simulink model "ALL_JP360_DBW_V6_5_1103"  (R2022a)
settings: Solver=FixedStepAuto  StartTime=0.0  StopTime=inf  FixedStep=0.01  RelTol=1e-3  EnableMultiTasking=on
model workspace (MAT data in the model file):
  g = 9.8
undefined symbols (not defined in the file or in its folder): canChannel, delta_v_p, IPM_Line_C0, IPM_Line_C1, IPM_Line_C2, IPM_Line_C3, M, M_p, MRR_ObjDistX, MRR_ObjDistY, MRR_ObjFusionCamID, MRR_ObjFusionSig, MRR_ObjID, MRR_ObjRelVelX, MRR_ObjRelVelY, MRR_ObjType, MRR_ObjUpdFlg, none, obj_vaild, untracktime, V, videoinput
libraries: canfdmsglib x230, canfdlib x76, slpidlib x24, simulink x18, dspstat3 x14, ctrlSharedLib x1, simulink_extras x1, imaqlib x1, realtime_pacer_lib x1, dspvision x1, visionsinks x1
(part 54 of 55)

== stateflow chart ALL_JP360_DBW_V6_5_1103/ACC_Control/ACC_FUNCTION/acc_stateflow/Chart2 ==
  settings: executeAtInitialization=1
  state total
    en:active_flg=0;set_flg=0;
    state a_set [parallel]
      settings: executionOrder=2
      state active
        state out
          en:set_speed_out=fcc(ABS_VehSpdLgt);
        state in
        state out_two
          en:set_speed_out=set_speed_in;
          du:set_speed_out=set_speed_in;
        (default) -> in
        in -> out [order 1] : [hasChangedFrom(SWM_ACCSet,0)]
        out -> out_two : [hasChangedFrom(SWM_ACCSet,0)||hasChangedFrom(SWM_ACCResume,0)]
        in -> out_two [order 2] : [hasChangedFrom(SWM_ACCResume,0)]
      state not_active
      state nomal_active
        du:set_speed_out=set_speed_in;
      not_active -> active [order 1] : [active_flg==1&&set_flg==1]
      (default) -> not_active
      active -> not_active : [active_flg~=1||set_flg~=1]
      nomal_active -> not_active : [active_flg==0]
      not_active -> nomal_active [order 2] : [active_flg==1&&set_flg==0]
    state acc [parallel]
      settings: executionOrder=1
      state NONE
      state INIT
        en:ACC_Status=0;flg=0;flg_quit=0;active_flg=0;
      note: set_resume=0:未激活
          | set_resume=1:按set激活
          | set_resume=2:按resume激活
      state AFTER_INIT
        state OFF
          en:ACC_Status=0;
          en:set_speed_out=0;
          en:flg=0;
          en:active_flg=0;set_flg=0;
        state STANDBY
          en:ACC_Status=2;
          en:active_flg=0;
        state PASSIVE
          en:ACC_Status=1;
          en:active_flg=0;
        state OVERRIDE
          en:ACC_Status=5;
          en:active_flg=0;
        state ACTIVE
          en:flg=flg+1;active_flg=1;
          state ACTIVE_CONTROL
            en:ACC_Status=3;
          state STAND_ACTIVE
            en:ACC_Status=6;
            en:three_s=1;
            en:flg_quit=flg_quit+1;
            du:flg_quit=flg_quit+1;
            state OFF
              y_stop=0;
            state ON
              en:y_stop=y_stop+1;
              du:y_stop=y_stop+1;
            (default) -> total.acc.AFTER_INIT.ACTIVE.STAND_ACTIVE.OFF
            total.acc.AFTER_INIT.ACTIVE.STAND_ACTIVE.OFF -> ON
          state STAND_WAIT
            en:ACC_Status=6;
            en:three_s=0;
            en:flg_quit=flg_quit+1;
            du:flg_quit=flg_quit+1;
          (default) -> ACTIVE_CONTROL
          STAND_WAIT -> ACTIVE_CONTROL [order 2] : [hasChangedFrom(SWM_ACCResume,1)&&EMS_BrkPedalStasus==0&&DriveOff==1&&SRS_SBR_Driver==0&&BCM_DoorStsFrntLe==1&&BCM_DoorStsFrntRi==1&&BCM_DoorStsRearLe==1&&BCM_DoorStsRearRi==1]{flg_quit=0}
          ACTIVE_CONTROL -> STAND_ACTIVE [order 1] : [ESP_VehicleStandstill==1&&SRS_SBR_Driver==0&&EMS_BrkPedalStasus==0&&DriveOff==0]
          STAND_ACTIVE -> ACTIVE_CONTROL [order 1] : [SRS_SBR_Driver==0&&EMS_BrkPedalStasus==0&&DriveOff==1]{flg_quit=0}
          STAND_ACTIVE -> STAND_WAIT [order 2] : [y_stop>=300]
          STAND_WAIT -> STAND_ACTIVE [order 1] : [hasChangedFrom(SWM_ACCResume,1)&&SRS_SBR_Driver==0&&EMS_BrkPedalStasus==0&&DriveOff==0]
        (default) -> total.acc.AFTER_INIT.OFF
        total.acc.AFTER_INIT.OFF -> STANDBY [order 2] : [hasChangedFrom(SWM_ACCSwitch,0)&&SWM_ACCSwitch~=2&&~(EMS_BrkPedalStasus==1||ESP_EPBStatus==1||ESP_EPBStatus==3||BCM_Mechanical_Hand_Brake==2||TCU_GearSelectorReq~=5||ABS_VehSpdDirection==1||BCM_DoorStsFrntLe==2||BCM_DoorStsFrntRi==2||BCM_DoorStsRearLe==2||BCM_DoorStsRearRi==2||BCM_EnginehoodSts==2||SRS_SBR_Driver==2)]
        STANDBY -> total.acc.AFTER_INIT.OFF [order 2] : [hasChangedFrom(SWM_ACCSwitch,0)&&SWM_ACCSwitch~=2]
        ACTIVE -> total.acc.AFTER_INIT.OFF [order 2] : [hasChangedFrom(SWM_ACCSwitch,0)&&SWM_ACCSwitch==2]{set_flg=0}
        total.acc.AFTER_INIT.OFF -> PASSIVE [order 1] : [hasChangedFrom(SWM_ACCSwitch,0)&&SWM_ACCSwitch~=2&&(EMS_BrkPedalStasus==1||ESP_EPBStatus==1||ESP_EPBStatus==3||BCM_Mechanical_Hand_Brake==2||TCU_GearSelectorReq~=5||ABS_VehSpdDirection==1||BCM_DoorStsFrntLe==2||BCM_DoorStsFrntRi==2||BCM_DoorStsRearLe==2||BCM_DoorStsRearRi==2||BCM_EnginehoodSts==2||SRS_SBR_Driver==2)]
        PASSIVE -> total.acc.AFTER_INIT.OFF [order 2] : [hasChangedFrom(SWM_ACCSwitch,0)&&SWM_ACCSwitch~=2]
        OVERRIDE -> total.acc.AFTER_INIT.OFF [order 3] : [hasChangedFrom(SWM_ACCSwitch,0)&&SWM_ACCSwitch==2]
        PASSIVE -> STANDBY [order 1] : [~(EMS_BrkPedalStasus==1||ESP_EPBStatus==1||ESP_EPBStatus==3||BCM_Mechanical_Hand_Brake==2||TCU_GearSelectorReq~=5||ABS_VehSpdDirection==1||BCM_DoorStsFrntLe==2||BCM_DoorStsFrntRi==2||BCM_DoorStsRearLe==2||BCM_DoorStsRearRi==2||BCM_EnginehoodSts==2||SRS_SBR_Driver==2)]
        (junction 53) -> PASSIVE
        STANDBY -> PASSIVE [order 1] : [EMS_BrkPedalStasus==1||ESP_EPBStatus==1||ESP_EPBStatus==3||BCM_Mechanical_Hand_Brake==2||TCU_GearSelectorReq~=5||ABS_VehSpdDirection==1||BCM_DoorStsFrntLe==2||BCM_DoorStsFrntRi==2||BCM_DoorStsRearLe==2||BCM_DoorStsRearRi==2||BCM_EnginehoodSts==2||SRS_SBR_Driver==2]
        (junction 140) -> (junction 53) : [(hasChangedFrom(SWM_ACCSwitch,0)&&SWM_ACCSwitch~=2)||ESP_EPBStatus==1||ESP_EPBStatus==3||BCM_Mechanical_Hand_Brake==2||TCU_GearSelectorReq~=5||ABS_VehSpdDirection==1||BCM_DoorStsFrntLe==2||BCM_DoorStsFrntRi==2||BCM_DoorStsRearLe==2||BCM_DoorStsRearRi==2||BCM_EnginehoodSts==2||SRS_SBR_Driver==2||flg_quit>=18000]{flg_quit=0,set_flg=0}
        ACTIVE_CONTROL -> (junction 53) [order 2] : [(hasChangedFrom(SWM_ACCSwitch,0)&&SWM_ACCSwitch~=2)||EMS_BrkPedalStasus==1||ESP_EPBStatus==1||ESP_EPBStatus==3||BCM_Mechanical_Hand_Brake==2||TCU_GearSelectorReq~=5||ABS_VehSpdDirection==1||BCM_DoorStsFrntLe==2||BCM_DoorStsFrntRi==2||BCM_DoorStsRearLe==2||BCM_DoorStsRearRi==2||BCM_EnginehoodSts==2||SRS_SBR_Driver==2]{set_flg=0}
        STANDBY -> ACTIVE [order 3] : [hasChangedFrom(SWM_ACCSet,0)&&~(EMS_BrkPedalStasus==1||ESP_EPBStatus==1||ESP_EPBStatus==3||BCM_Mechanical_Hand_Brake==2||TCU_GearSelectorReq~=5||ABS_VehSpdDirection==1||BCM_DoorStsFrntLe==2||BCM_DoorStsFrntRi==2||BCM_DoorStsRearLe==2||BCM_DoorStsRearRi==2||BCM_EnginehoodSts==2||SRS_SBR_Driver==2)&&(EMS_AccRAWPedalRatio==0||EMS_AccRAWPedalRatio==255)]{set_speed_out=fcc(ABS_VehSpdLgt)}
        STANDBY -> ACTIVE [order 4] : [(hasChangedFrom(SWM_ACCResume,0)&&flg~=0)&&~(EMS_BrkPedalStasus==1||ESP_EPBStatus==1||ESP_EPBStatus==3||BCM_Mechanical_Hand_Brake==2||TCU_GearSelectorReq~=5||ABS_VehSpdDirection==1||BCM_DoorStsFrntLe==2||BCM_DoorStsFrntRi==2||BCM_DoorStsRearLe==2||BCM_DoorStsRearRi==2||BCM_EnginehoodSts==2||SRS_SBR_Driver==2)&&(EMS_AccRAWPedalRatio==0||EMS_AccRAWPedalRatio==255)]
        OVERRIDE -> PASSIVE [order 2] : [(hasChangedFrom(SWM_ACCSwitch,0)&&SWM_ACCSwitch~=2)||EMS_BrkPedalStasus==1||ESP_EPBStatus==1||ESP_EPBStatus==3||BCM_Mechanical_Hand_Brake==2||TCU_GearSelectorReq~=5||ABS_VehSpdDirection==1||BCM_DoorStsFrntLe==2||BCM_DoorStsFrntRi==2||BCM_DoorStsRearLe==2||BCM_DoorStsRearRi==2||BCM_EnginehoodSts==2||SRS_SBR_Driver==2]
        OVERRIDE -> ACTIVE [order 1] : [EMS_IndicatedDriverOverride==0]{set_flg=1}
        ACTIVE -> OVERRIDE [order 1] : [EMS_IndicatedDriverOverride==1]{set_flg=0}
        STAND_WAIT -> (junction 140) [order 3]
        STAND_ACTIVE -> (junction 140) [order 3]
      state FALURE_REVERSIBLE
        en:ACC_Status=7;
        en:active_flg=0;
      state FALURE_IRREVERSIBLE
        en:ACC_Status=7;
        en:active_flg=0;
      (default) -> NONE
      NONE -> INIT : [BCM_PowerModeInvalid==0&&BCM_PowerMode==2&&ESP_EspEnableSts==1&&EPS_EPSPAMSts~=7&&EMS_IndicatedEngError==0&&MRR_HWFail==0&&IPM_SensorState==0]
      INIT -> AFTER_INIT
      AFTER_INIT -> FALURE_REVERSIBLE [order 1] : [acc_state_sw==1]
      FALURE_REVERSIBLE -> AFTER_INIT [order 1] : [acc_state_sw==0]
      FALURE_REVERSIBLE -> FALURE_IRREVERSIBLE [order 2] : [acc_state_sw==2||ESP_EspEnableSts==0||EPS_EPSPAMSts==7||EMS_IndicatedEngError==1||MRR_HWFail==1||IPM_SensorState==4]
      AFTER_INIT -> FALURE_IRREVERSIBLE [order 2] : [acc_state_sw==2||ESP_EspEnableSts==0||EPS_EPSPAMSts==7||EMS_IndicatedEngError==1||MRR_HWFail==1||IPM_SensorState==4]
  data: y function_output; VehSpdLgt function_input; SWM_ACCSwitch input; SWM_ACCSet input; SWM_ACCResume input; BCM_DoorStsFrntLe input; BCM_DoorStsFrntRi input; BCM_DoorStsRearLe input; BCM_DoorStsRearRi input; BCM_PowerModeInvalid input; BCM_PowerMode input; BCM_Mechanical_Hand_Brake input; BCM_EnginehoodSts input; IPM_SensorState input; MRR_HWFail input; SRS_SBR_Driver input; EMS_IndicatedEngError input; EMS_AccRAWPedalRatio input; EMS_BrkPedalStasus input; EPS_EPSPAMSts input; TCU_GearSelectorReq input; ESP_EPBStatus input; ESP_EspEnableSts input; ABS_VehSpdDirection input; ESP_AvhActive input; ESP_VehicleStandstill input; DriveOff input; acc_state_sw input; ACC_Status output int8; flg local; set_speed_in input; ABS_VehSpdLgt input; EMS_IndicatedDriverOverride input; set_speed_out output uint8; three_s output; y_stop local; flg_quit local; active_flg local; set_flg local
  function y=fcc(VehSpdLgt):
    | function y=fcc(VehSpdLgt)
    |  
    | if VehSpdLgt <=uint8(30)
    |     y=uint8(30);
    | else
    |     y=VehSpdLgt;
    | end
    | 
    | end

== matlab function ALL_JP360_DBW_V6_5_1103/ACC_Control/ACC_FUNCTION/Subsystem2/Limit/a2m_表达式_标定表/MATLAB Function ==
  data: delta_v input; y output; p1 input; p2 input
function y = fcn(delta_v,p1,p2)
    if delta_v < 1 && delta_v > -0.05
        y = single(p1);
    elseif delta_v <=-0.05
        y = single(p2);
    else
        y=single(0);
    end
end

== matlab function ALL_JP360_DBW_V6_5_1103/ACC_Control/ACC_FUNCTION/Subsystem2/ACC_model/CC_module/MATLAB Function ==
  data: acc_in input; delta_v input; acc_out output; dec_in input; dec_out output
function [acc_out, dec_out] = fcn(acc_in,delta_v, dec_in)
    if delta_v > -2.5
        acc_out = acc_in;
%         if delta_v >-0.1
%             dec_out = single(0);
%         else
%             if dec_in < 0
%                 dec_in = dec_in + single(0.05);
%                 dec_out = dec_in;
%             else
                dec_out = single(0);
%             end
%         end
    else
        acc_out = single(0);
        dec_out = dec_in;
    end
end

== matlab function ALL_JP360_DBW_V6_5_1103/ACC_Control/ACC_FUNCTION/Subsystem2/Limit/MATLAB Function ==
  data: u input; y1 output; data input; y2 output
function [y1,y2] = fcn(u, data)
%此函数的功能为：当err_v在(-1,0)时，输出-10nm；(-2,-1)时，输出扭矩-30nm；
%err_v小于等于-2时，输出PID计算的减速度；
y1=single(0);
y2=single(0);
if -1<u&&u<0
    y1=single(-10);
elseif -2<u&&u<=-1
    y1=single(-30);
elseif u<=-2
    y2=single(data);
else
    y1=single(0);
    y2=single(0);
end

== stateflow chart ALL_JP360_DBW_V6_5_1103/button/ACCset/ACC_button/Subsystem4/Chart1 ==
  state ON
    en:y=y+t;
    du:y=y+t;
  state OFF
    y=0;
  (default) -> (junction 1)
  (junction 1) -> OFF [order 2]
  (junction 1) -> ON [order 1] : [u1==3]
  OFF -> ON : [u1==3]
  ON -> OFF : [u1~=3]
  data: y output uint16; t input uint16; u1 input int8

== stateflow chart ALL_JP360_DBW_V6_5_1103/DCLC1/DCLC状态机/Chart1 ==
  state OFF
    en:
    count = 0;
  state ON
    en:
    count = count + 1;
    du:
    count = count + 1;
  (default) -> OFF
  OFF -> ON : [condition == 1]
  ON -> OFF : [condition == 0]
  data: condition input; count output

== stateflow chart ALL_JP360_DBW_V6_5_1103/ACC_Control/ACC_FUNCTION/Subsystem2/override/Chart2 ==
  settings: executeAtInitialization=1
  state ON
  state OFF
  (default) -> OFF
  OFF -> ON : status{u1=1}
  ON -> OFF : mode{u1=0}
  data: u1 output
  events: status input EITHER_EDGE_EVENT; mode input EITHER_EDGE_EVENT

== matlab function ALL_JP360_DBW_V6_5_1103/DCLC1/AngleSaftyLimitedCal ==
  data: a input single; angle_limited output single; L input single; V input single; angle input single
function angle_limited= fcn(a,L,V,angle)
if abs(V) > 19.5
    a = single(0.8);
end
angle_max = atan(a*L/V/V)*16*57.3;
if angle > angle_max
    angle_limited = angle_max;
elseif angle < -angle_max
        angle_limited = -angle_max;
else
    angle_limited = angle;
end

if angle_limited > single(20)
    angle_limited = single(20);
elseif angle_limited < -20
    angle_limited = single(-20);
end

end

== matlab function ALL_JP360_DBW_V6_5_1103/LKA_Control/LKA_Cal/LKAControlerl/MATLAB Function ==
  data: LKA_status input int8; err input; ang_rate output single; LKA_sta data_store_memory; t_ca data_store_memory; sta_change data_store_memory
function ang_rate = fcn(LKA_status,err)

global LKA_sta;
global t_ca;
global sta_change;

if LKA_sta==1 && LKA_status ==4
    sta_change = int8(1);
end
if LKA_status ==4 && sta_change == 1
    t_ca = t_ca +int8(1);
    ang_rate = single(2);
    if err <0.15 || t_ca >300
        sta_change = int8(0);
        t_ca = int8(0);
        ang_rate = single(25);
    end
else
    sta_change = int8(0);
    t_ca =int8(0);
    ang_rate = single(25);
end

end

== stateflow chart ALL_JP360_DBW_V6_5_1103/button/ACCset/ACC_button/Subsystem4/Chart2 ==
  state init
    state ON
      y=true;
    state OFF
      y=false;
    init -> (junction 1)
    (default) -> (junction 1)
    (junction 1) -> OFF [order 2]
    (junction 1) -> ON [order 1] : [u1>=20]
  (default) -> init
  data: y output boolean; u1 input uint16

== stateflow chart ALL_JP360_DBW_V6_5_1103/button/ACCset/ACC_button/Subsystem3/Chart ==
  state ON
    en:y=y+t;
    du:y=y+t;
  state OFF
    y=0;
  (default) -> (junction 1)
  (junction 1) -> OFF [order 2]
  (junction 1) -> ON [order 1] : [u1==1]
  OFF -> ON : [u1==1]
  ON -> OFF : [u1==0]
  data: y output uint16; t input; u1 input

== stateflow chart ALL_JP360_DBW_V6_5_1103/button/ACCset/ACC_button/Subsystem3/Chart10 ==
  state init
    state ON1
      en:y=1;
    state ON
      en:y=floor(u1/80)+1;
    state OFF
      y=0;
    init -> (junction 1)
    (default) -> (junction 1)
    (junction 1) -> OFF [order 3]
    (junction 1) -> ON [order 1] : [u1>=80]
    (junction 1) -> ON1 [order 2] : [u1>=4&&u1<80]
  (default) -> init
  data: y output single; u1 input single

== stateflow chart ALL_JP360_DBW_V6_5_1103/button/ACCset/ACC_button/accsetv2 ==
  state s1
    speedout=false;
  state s
    speedout=speed;
  (default) -> s1
  s1 -> s : [accs==3]
  s -> s1 : [accs~=3]
  data: speedout output boolean; accs input; speed input boolean

== stateflow chart ALL_JP360_DBW_V6_5_1103/button/ACCset/ACC_button/Subsystem1/Chart ==
  state ON
    en:y=y+t;
    du:y=y+t;
  state OFF
    y=0;
  (default) -> (junction 1)
  (junction 1) -> OFF [order 2]
  (junction 1) -> ON [order 1] : [u1==1]
  OFF -> ON : [u1==1]
  ON -> OFF : [u1==0]
  data: y output uint16; t input; u1 input

== stateflow chart ALL_JP360_DBW_V6_5_1103/button/ACCset/ACC_button/Subsystem1/Chart10 ==
  state init
    state ON1
      en:y=1;
    state ON
      en:y=fix(u1/80)+1;
    state OFF
      y=0;
    init -> (junction 1)
    (default) -> (junction 1)
    (junction 1) -> OFF [order 3]
    (junction 1) -> ON [order 1] : [u1>=80]
    (junction 1) -> ON1 [order 2] : [u1>=4&&u1<80]
  (default) -> init
  data: y output single; u1 input single

== stateflow chart ALL_JP360_DBW_V6_5_1103/button/ACCset/ACC_button/accsetv1 ==
  state s1
    speedout=false;
  state s
    speedout=speed;
  (default) -> s1
  s1 -> s : [accs==3]
  s -> s1 : [accs~=3]
  data: speedout output boolean; accs input; speed input boolean

== stateflow chart ALL_JP360_DBW_V6_5_1103/button/ACCset/ACC_button/Chart1 ==
  state s
    state start1
      a=speed;
    state pluss
      en:a=floor(speed/10)*10+10;
    state pluss1
      en:a=speed+1;
    state minn1
      en:a=ceil(speed/10)*10-10;
    state minn
      en:a=speed-1;
    s -> (junction 54)
    (default) -> start1
    (junction 54) -> start1 [order 5]
    (junction 54) -> minn [order 3] : [min==1]
    (junction 54) -> minn1 [order 1] : [min>=2]
    (junction 54) -> pluss [order 2] : [plus>=2]
    (junction 54) -> pluss1 [order 4] : [plus==1]
  (default) -> s
  data: a output; plus input; min input; speed input
  events: event input RISING_EDGE_EVENT

== stateflow chart ALL_JP360_DBW_V6_5_1103/button/ACCset/ACC_button/Chart2 ==
  state s
    state s
    state pluss1
      speedout=150;
    state minn1
      speedout=30;
    state minn
      speedout=speed;
    state minn2 [commented out]
      speedout=0;
    s -> (junction 54)
    (default) -> s.s
    (junction 54) -> s.s [order 4]
    (junction 54) -> minn [order 2] : [speed>=30&&speed<=150]
    (junction 54) -> minn2 [commented out] : [speed==0]
    (junction 54) -> minn1 [order 1] : [speed<=30&&speed>=0]
    (junction 54) -> pluss1 [order 3] : [speed>150]
  (default) -> s
  data: speedout output uint8; speed input

== stateflow chart ALL_JP360_DBW_V6_5_1103/button/ACCset/ACC_button/Subsystem2/Chart ==
  state ON
    en:y=y+t;
    du:y=y+t;
  state OFF
    y=0;
  (default) -> (junction 1)
  (junction 1) -> OFF [order 2]
  (junction 1) -> ON [order 1] : [u1==1]
  OFF -> ON : [u1==1]
  ON -> OFF : [u1==0]
  data: y output uint16; t input; u1 input

== stateflow chart ALL_JP360_DBW_V6_5_1103/button/ACCset/ACC_button/Subsystem2/Chart10 ==
  state init
    state ON1
      en:y=1;
    state ON
      en:y=fix(u1/80)+1;
    state OFF
      y=0;
    init -> (junction 1)
    (default) -> (junction 1)
    (junction 1) -> OFF [order 3]
    (junction 1) -> ON [order 1] : [u1>=80]
    (junction 1) -> ON1 [order 2] : [u1>=4&&u1<80]
  (default) -> init
  data: y output uint16; u1 input uint16

== matlab function ALL_JP360_DBW_V6_5_1103/DCLC1/DCLC planner/change lane ==
  data: status output int16 size=1; dclc_sts input int8; width output single size=1; c0 input single size=4; c1 input single size=4; heading output single; diff_y output single; turn_request input int8
function [status, width, heading, diff_y] = fcn(dclc_sts, c0, c1, turn_request)
persistent change_state; %是否变道线
if isempty(change_state) 
    change_state = boolean(0);
end
% timeposition = time_position;
% global pre_position;
% if isempty(pre_position) 
%     pre_position = int32(1);
% end
% global left_buf;
% global right_buf;
% last_state = -1;
% persistent left_buf;
% persistent right_buf;
% persistent width_togo;
% 
% if isempty(left_buf) 
%     left_buf = single(0.0);
% end
% if isempty(right_buf) 
%     right_buf = single(0.0);
% end
% if isempty(width_togo) 
%     width_togo = single(0.0);
% end

% left_finish = 0;
% right_finish = 0;
% left_back_finish = 0;
% right_back_finish = 0;
% reach_dest = 0;
% time_count = 0;

% c1 左左车道线到自车的横向距离
% c2 左车道线到自车的横向距离
% c3 右车道线到自车的横向距离
% c4 右右车道线到自车的横向距离

% if (dclc_sts_last == 21) && (dclc_sts == 22)        % 左变道开始
%     left_buf = Y0;
%     width_togo = c0(2) + (c0(1) - c0(2)) / 2;
%     width = width_togo + left_buf - Y0;
%     heading = c1(2);
%     status = 1;
%     time_count = 0;
% elseif (dclc_sts_last == 31) && (dclc_sts == 32)    % 右变道开始
%     right_buf = Y0;
%     width_togo = c0(3) + (c0(4) - c0(3)) / 2;
%     width = width_togo + right_buf - Y0;
%     heading = c1(3);
%     status = 1;
%     time_count = 0;
% elseif (dclc_sts_last == 22) && (dclc_sts == 23)    % 左变道回退
%     right_buf = Y0;
%     width_togo = c0(2) + (c0(3) - c0(2)) / 2;
%     width = width_togo + right_buf - Y0;
%     heading = c1(2);
%     status = 1;
%     time_count = 0;
% elseif (dclc_sts_last == 32) && (dclc_sts == 33)    % 右变道回退
%     left_buf = Y0;
%     width_togo = c0(3) + (c0(2) - c0(3)) / 2;
%     width = width_togo + left_buf - Y0;
%     heading = c1(3);
%     status = 1;
%     time_count = 0;
% elseif (dclc_sts == 22) || (dclc_sts == 33)         % 左变道中 / 右变道回退
%     width = width_togo + left_buf - Y0;
%     heading = c1(2);
%     if (abs(width) < 0.1) && (count < 2000)         % 加入持续时间判断
%         time_count = count + 1;
%     elseif (abs(width) < 0.1) && (count >= 2000)  
%         time_count = count;
%         reach_dest = 1;
%     end
%     status = 1;
% elseif (dclc_sts == 32) || (dclc_sts == 23)         % 右变道中 / 左变道回退
%     width = width_togo + right_buf - Y0;
%     heading = c1(3);
%     if (abs(width) < 0.1) && (count < 2000)         % 加入持续时间判断
%         time_count = count + 1;
%     elseif (abs(width) < 0.1) && (count >= 2000)  
%         time_count = count;
%         reach_dest = 1;
%     end
%     status = 1;
% else
%     status = 0;  %其他状态
%     width = 0;
%     heading = 0;
%     time_count = 0;
% end
diff_y = single(0);
if dclc_sts == int8(22)   % 左变道中
    if c0(2) > single(3.0)
        change_state = boolean(1);
    end
    heading = c1(2);
    if change_state
        width = c0(2) - (c0(2) - c0(3))/2;
%         heading = c1(2);
        status = int16(2);
        if turn_request == int8(0)
            status =  int16(4);
        end
    else
        width = c0(2) + (c0(1) - c0(2)) / 2;
        diff_heading = atan(heading);
        diff_y = sin(diff_heading) * 6.5 - cos(diff_heading)*1;
        if -diff_y > c0(2)
            status = int16(4);
        else
            status = int16(3);
        end
    end
elseif dclc_sts == int8(32)    % 右变道中
    if c0(3) < single(-3.0)
        change_state = boolean(1);
    end
    heading = c1(3);
    if change_state
        width = c0(3) + (c0(2) - c0(3)) / 2;
%         heading = c1(3);
        status = int16(2);
        if turn_request == int8(0)
            status =  int16(4);
        end
    else
        width = c0(3) + (c0(4) - c0(3)) / 2;
        diff_heading = atan(heading);
        diff_y = sin(diff_heading) * 6.5 + cos(diff_heading)*1;
        if -diff_y < c0(3)
            status = int16(4);
        else
            status = int16(3);
        end
    end
elseif dclc_sts == int8(23)   %左回退
    width = c0(2) + (c0(3) - c0(2)) / 2;
    heading = c1(2);
    status = int16(1);
%     if time_position ~= int32(1)
%         timeposition = int32(1);
%     end
elseif dclc_sts == int8(33)   %右回退
    width = c0(3) + (c0(2) - c0(3)) / 2;
    heading = c1(3);
    status = int16(1);
%     if time_position ~= int32(1)
%         timeposition = int32(1);
%     end
else
    status = int16(0);  %其他状态
    width = single(0);
    heading = single(0);
    change_state = boolean(0);
%     timeposition = int32(1);
end

end

== matlab function ALL_JP360_DBW_V6_5_1103/DCLC1/DCLC planner/error_compute ==
  data: xrr output single size=1; yrr output single size=1; thetarr output single size=1; krr output single size=1; start_position input int32; width input single; status input int8; heading input; diff_y input; diff_x input
 % function [xrr,yrr,thetarr,krr,k_d] = fcn(x,y,xr,yr,thetar,kappar)
% n = length(xr);
%    %d_min = (x-xr(1))^2 + (y-yr(1))^2; % 根据距离最近原则计算预瞄位置与参考轨迹上连线距离最近点的距离,这只是一个初始值
%    e_min=1;
%    k_d=1;
%    %kend=k+50;
% %    if kend >= n
% %        kend=n;
% %    end
%    %for i = k+1:kend                                 % 遍历参考轨迹上的所有的点，i为点的索引值
%    for i = 1:n
%        d = sqrt((x-xr(i))^2 + (y-yr(i))^2);       % 在大地坐标系下的欧氏距离
%        if d < e_min
%            e_min = d;
%            k_d = i;                               % 根据最短欧式距离获取匹配点的索引值
%        end
%    end
%    xrr=xr(k_d);
%    yrr=yr(k_d);
%    thetarr=thetar(k_d);
%    krr=kappar(k_d);
%    %arr=ar(k_d);
%    %vrr=vr(k_d);
% end

function [xrr,yrr,thetarr,krr] = fcn(start_position, width, status, heading, diff_y, diff_x)
%     global pre_position;
%   persistent x_position;
%   persistent y_position;
% 
%   if isempty(x_position) 
%       x_position = single(0);
%   end
% 
%   if isempty(y_position) 
%       y_position = single(0);
%   end
%     n = length(xr);
    if status == int8(22) || status == int8(33) || status == int8(32) || status == int8(23)
        yrr = width - diff_y;
        thetarr = heading;
    else
        yrr = single(0);
        thetarr = single(0);
    end

    xrr = single(0);
    krr = single(0);
%     timeposition = int32(1);
    
%     w_cur = yr(n) - width;
%     target_position = int32(1);
%     head = single(0);
%     indix = int32(1);
%     diff = single(1e5);
% %     target_position = start_position;
%     if status == int8(22) || status == int8(33)
%         x_position = x_position + diff_x;
%         y_position = y_position + diff_y;
%         for i=time_position:n
%             distance = (x_position - xr(i))*(x_position - xr(i)) + (y_position - yr(i))*(y_position - yr(i));
%             if distance <= diff
%                 indix = int32(i);
%                 diff = distance;
%                 head = heading;
%                % break;
%             end
%         end
% %         position = int32(find(yr > w_cur, 1));
%     elseif status == int8(32) || status == int8(23)
%         x_position = x_position + diff_x;
%         y_position = y_position + diff_y;
%         for i=time_position:n
%             distance = (x_position - xr(i))*(x_position - xr(i)) + (y_position - yr(i))*(y_position - yr(i));
%             if distance <= diff
%                 indix = int32(i);
%                 diff = distance;
%                 head = heading;
%                % break;
%             end
%         end
% %         position = int32(find(yr < w_cur, 1));
%     else
%         x_position = single(0);
%         y_position = single(0);
%     end
% 
% %     if cur_position <= time_position
% %         cur_position = cur_position + 1;
% %     end
% % 滑动窗口
%     target_position = min(n, (indix + start_position));
% 
% %     time_position = int32(min(n, time_position+1));
% 
% %     position = max(cur_position, pre_position+1);
% %     if position == int32(0)
% %         position = int32(n);
% %         target_position = position;
% %     else
% %         target_position = position + start_position;
% %     end
% %     while position < n && abs(yr(pre_position)) < 1e-4
% %           position = position + pre_position;
% %     end
%     xrr=xr(target_position) - xr(indix);
% %     yrr=yr(target_position) - y_position;
%      yrr=yr(target_position) - yr(indix);
%     if indix == n
%         yrr = width;
%     end
% %     yrr=yr(target_position) - y_position;
%     thetarr=single(thetar(target_position) + head);
%     krr=kappar(target_position);
%       preposition = int32(position);

%     if n >= target_position
%         xrr=xr(target_position) - xr(position);
%         yrr=yr(target_position) - yr(position);
%         thetarr=thetar(target_position) - thetar(position);
%         krr=kappar(target_position) - kappar(position);
%         preposition = int32(position);
%     else
%         xrr=xr(n) - xr(position);
%         yrr=yr(n) - yr(position);
%         thetarr=thetar(n) - thetar(position);
%         krr=kappar(n) - kappar(position);
%         preposition = int32(n);
%     end
%     timeposition = indix;
end





% function [xrr,yrr,thetarr,krr,dmin] = fcn(x_rear,y_rear,xr,yr,thetar,kappar)
% n = length(xr);
%     d_min = (x_rear-xr(1))^2 + (y_rear-yr(1))^2; % 根据距离最近原则计算预瞄位置与参考轨迹上连线距离最近点的距离,这只是一个初始值
%     min = 1;
%     for i = 1:n                                  % 遍历参考轨迹上的所有的点，i为点的索引值
%         d = (x_rear-xr(i))^2 + (y_rear-yr(i))^2; %在大地坐标系下的欧氏距离
%         if d < d_min
%         d_min = d;
%         min = i;                             % 根据最短欧式距离获取匹配点的索引值
%         end
%     end
%     dmin = min;
%     xrr=xr(dmin);
%     yrr=yr(dmin);
%     thetarr=thetar(dmin);
%     krr=kappar(dmin);
% end

== matlab function ALL_JP360_DBW_V6_5_1103/DCLC1/DCLC planner/width compute ==
  data: u input single; y output single; status input int16; change_end_status output single; heading input
function [y, change_end_status]  = fcn(u, status, heading)

change_end_status = single(0);

if abs(u) <= 0.2
   if(status)
       if abs(heading) < 0.025
           change_end_status = single(1);
           %time_count = single(200);
       end
   end
   y = single(0);
%    time_count = single(0);
elseif (status == 1) && (abs(u) <= 0.4)
    change_end_status = single(1);
    y = single(0);
else
   y = u;
end

== stateflow chart ALL_JP360_DBW_V6_5_1103/DCLC1/DCLC状态机/Chart ==
  state DCLC_OFF
    du:DCLC_sts=int8(0);
  state DCLC_ON
    state STANDBY
      state Inhibit
        du:DCLC_sts=int8(10);
      state Enable
        state Enable_left
          du:DCLC_sts=int8(11);
        state Enable_right
          du:DCLC_sts=int8(12);
        state Enable_both
          du:DCLC_sts=int8(13);
        Enable_left -> Enable_right [order 1] : [((left_lane_line_clear ~= 1) && (right_lane_line_clear == 1)) || ((IPM_RightLine_Type == 3) && (IPM_LeftLine_Type ~= 3))]
        Enable_right -> Enable_left [order 1] : [((left_lane_line_clear == 1) && (right_lane_line_clear ~= 1)) || ((IPM_LeftLine_Type == 3) && (IPM_RightLine_Type ~= 3))]
        Enable_both -> Enable_left [order 1] : [((left_lane_line_clear == 1) && (right_lane_line_clear ~= 1)) || ((IPM_LeftLine_Type == 3) && (IPM_RightLine_Type ~= 3))]
        Enable_left -> Enable_both [order 2] : [(left_lane_line_clear == 1) && (right_lane_line_clear == 1) && (IPM_LeftLine_Type == 3) && (IPM_RightLine_Type == 3)]
        (junction 43) -> Enable_left [order 1] : [((left_lane_line_clear == 1) && (right_lane_line_clear ~= 1)) || ((IPM_LeftLine_Type == 3) && (IPM_RightLine_Type ~= 3))]
        (junction 43) -> Enable_right [order 2] : [((left_lane_line_clear ~= 1) && (right_lane_line_clear == 1)) || ((IPM_LeftLine_Type ~= 3) && (IPM_RightLine_Type == 3))]
        Enable_right -> Enable_both [order 2] : [(left_lane_line_clear == 1) && (right_lane_line_clear == 1) && (IPM_LeftLine_Type == 3) && (IPM_RightLine_Type == 3)]
        Enable_both -> Enable_right [order 2] : [((left_lane_line_clear ~= 1) && (right_lane_line_clear == 1)) || ((IPM_LeftLine_Type ~= 3) && (IPM_RightLine_Type == 3))]
        (default) -> (junction 43)
        (junction 43) -> Enable_both [order 3]
      (default) -> Inhibit
      Inhibit -> Enable : [(ACC_Enable == 1) && (LKA_Enable == 1) && (BCM_TurnIndicatorDig == 0) && (IPM_SensorState == 0) && (FLR_SRR_Obj_Failure == 0) && (FRR_SystemStatus ~= 7) && (RRR_SystemStatus ~= 7) && (RLR_SRR_Obj_Failure == 0) &&(ADU1_TurnLightReq == 0) && ((left_lane_line_clear == 1) || (right_lane_line_clear == 1)) && ((IPM_LeftLine_Type == 3) || (IPM_RightLine_Type == 3))]
      Enable -> Inhibit : [(ACC_Enable ~= 1) || (LKA_Enable ~= 1) || ((left_lane_line_clear ~= 1) && (right_lane_line_clear ~= 1)) || (BCM_TurnIndicatorDig == 1) || (IPM_SensorState == 4) || (FLR_SRR_Obj_Failure == 1) || (FRR_SystemStatus == 7) || (RRR_SystemStatus == 7) || (RLR_SRR_Obj_Failure == 1) || ((IPM_LeftLine_Type ~= 3) && (IPM_RightLine_Type ~= 3))]
    state ACTIVE
      state ACTIVE_L
        state WAIT_L
          du:DCLC_sts=int8(21);
        state MOVING_L
          du:DCLC_sts=int8(22);
        state END_L
          du:DCLC_sts=int8(24);
        state RETURN_L
          du:DCLC_sts=int8(23);
        (default) -> WAIT_L
        WAIT_L -> MOVING_L [order 1] : [((MRR_F_Object_dist > Front_Distance_Threshold) && (FLR_OBJ1_Dist > Left_Front_Distance_Threshold) && (RLR_OBJ1_Dist > Left_Rear_Distance_Threshold) && (IPM_LeftLine_Color == 1) && (IPM_LeftLine_Type == 3) && (ABS_VehSpdLgt > Speed_Min + 2) && (ABS_VehSpdLgt < Speed_Max - 10) && (IPM_LeftLine_dy > Left_Line_Width_Threshold) && (IPM_RightLine_dy < Right_Line_Width_Threshold) && (IPM_LeftLine_hor_curve < Curve_Threshold) && (BCM_TurnIndicatorDig == 0) && (EPS2_EPS1TASTrq > Negative_Torque) && (EPS2_EPS1TASTrq < Positive_Torque) && (IPM_SensorState == 0) && (FLR_SRR_Obj_Failure == 0) && (FRR_SystemStatus ~= 7) && (RRR_SystemStatus ~= 7) && (RLR_SRR_Obj_Failure == 0) && (~MRR_HWFail) && after(K_LCD_Wait_Time_Low, sec) && before(K_LCD_Wait_Time_Upper, sec)) ]
        WAIT_L -> END_L [order 2] : [(after(K_LCD_Wait_Time_Upper, sec) || (EPS2_EPS1TASTrq < Negative_Torque) || (ADU1_TurnLightReq == 0) || (ABS_VehSpdLgt > Speed_Max) || (ABS_VehSpdLgt < Speed_Min))]
        MOVING_L -> END_L [order 2] : [(Reach_Destination == 1) || ((Pass_Midline == 2) && (ADU1_TurnLightReq == 0))]
        MOVING_L -> RETURN_L [order 1] : [ (Pass_Midline == 3) && ((ADU1_TurnLightReq == 0) || (ADU1_TurnLightReq == 2) || (ABS_VehSpdLgt < Speed_Min) || (ABS_VehSpdLgt > Speed_Max) ||  (FLR_OBJ1_Dist < Left_Front_Distance_Threshold) || (RLR_OBJ1_Dist < Left_Rear_Distance_Threshold) || (EPS2_EPS1TASTrq < Negative_Torque) || (FLR_SRR_Obj_Failure == 1) || (FRR_SystemStatus == 7) || (RRR_SystemStatus == 7) || (RLR_SRR_Obj_Failure == 1))]
        RETURN_L -> END_L : [Reach_Destination == 1]
      state ACTIVE_R
        state MOVING_R
          du:DCLC_sts=int8(32);
        state WAIT_R
          du:DCLC_sts=int8(31);
        state RETURN_R
          du:DCLC_sts=int8(33);
        state END_R
          du:DCLC_sts=int8(34);
        (default) -> WAIT_R
        WAIT_R -> MOVING_R [order 1] : [[(MRR_F_Object_dist > Front_Distance_Threshold) && (FRR_OBJ1_Dist > Right_Front_Distance_Threshold) &&(RRR_OBJ1_Dist > Right_Rear_Distance_Threshold) && (IPM_RightLine_Color == 1) && (IPM_RightLine_Type == 3) && (ABS_VehSpdLgt > Speed_Min + 2) && (ABS_VehSpdLgt < Speed_Max - 10) && (IPM_LeftLine_dy > Left_Line_Width_Threshold) && (IPM_RightLine_dy < Right_Line_Width_Threshold) && (IPM_RightLine_hor_curve < Curve_Threshold) && (BCM_TurnIndicatorDig == 0) && (EPS2_EPS1TASTrq > Negative_Torque) && (EPS2_EPS1TASTrq < Positive_Torque) && (IPM_SensorState == 0) && (FLR_SRR_Obj_Failure == 0) && (FRR_SystemStatus ~= 7) && (RRR_SystemStatus ~= 7) && (RLR_SRR_Obj_Failure == 0) && (~MRR_HWFail) && after(K_LCD_Wait_Time_Low, sec) && before(K_LCD_Wait_Time_Upper, sec)]]
        MOVING_R -> RETURN_R [order 1] : [(Pass_Midline == 3) && ((ADU1_TurnLightReq == 0) || (ADU1_TurnLightReq == 1) || (ABS_VehSpdLgt > Speed_Max) || (ABS_VehSpdLgt < Speed_Min) ||  (FRR_OBJ1_Dist < Right_Front_Distance_Threshold) || (RRR_OBJ1_Dist < Right_Rear_Distance_Threshold) || (EPS2_EPS1TASTrq > Positive_Torque) || (FLR_SRR_Obj_Failure == 1) || (FRR_SystemStatus == 7) || (RRR_SystemStatus == 7) || (RLR_SRR_Obj_Failure == 1))]
        MOVING_R -> END_R [order 2] : [(Reach_Destination == 1) || ((Pass_Midline == 2) && (ADU1_TurnLightReq == 0))]
        WAIT_R -> END_R [order 2] : [after(K_LCD_Wait_Time_Upper, sec) || (EPS2_EPS1TASTrq > Positive_Torque) || (ADU1_TurnLightReq == 0) || (ABS_VehSpdLgt > Speed_Max) || (ABS_VehSpdLgt < Speed_Min)]
        RETURN_R -> END_R : [Reach_Destination == 1]
      WAIT_L -> ACTIVE_R [order 3] : [(ADU1_TurnLightReq == 2) && (BCM_TurnIndicatorDig ==0)]
      WAIT_R -> ACTIVE_L [order 3] : [(ADU1_TurnLightReq == 1) && (BCM_TurnIndicatorDig ==0)]
    (default) -> STANDBY
    Enable_left -> ACTIVE_L [order 3] : [(ADU1_TurnLightReq == 1) && (BCM_TurnIndicatorDig == 0) && (IPM_SensorState == 0) && (FLR_SRR_Obj_Failure == 0) && (FRR_SystemStatus ~= 7) && (RRR_SystemStatus ~= 7) && (RLR_SRR_Obj_Failure == 0)]
    Enable_right -> ACTIVE_R [order 3] : [(ADU1_TurnLightReq == 2) && (BCM_TurnIndicatorDig == 0) && (IPM_SensorState == 0) && (FLR_SRR_Obj_Failure == 0) && (FRR_SystemStatus ~= 7) && (RRR_SystemStatus ~= 7) && (RLR_SRR_Obj_Failure == 0)]
    END_L -> STANDBY : [after(t_planning, sec) && (ADU1_TurnLightReq == 0) ]
    END_R -> STANDBY : [(after(t_planning, sec)) && (ADU1_TurnLightReq == 0) ]
    ACTIVE -> STANDBY : [(ACC_Enable ~= 1) || (LKA_Enable ~= 1) || ((EPS2_EPS1TASTrq > Positive_Torque) && after(K_SACC_Override_Time, sec)) || ((EPS2_EPS1TASTrq < Negative_Torque) && after(K_SACC_Override_Time, sec)) || ((ADU1_LongCtrlMode == 1) && after(K_SACC_Override_Time, sec))]
    Enable_both -> ACTIVE_L [order 3] : [(ADU1_TurnLightReq == 1) && (BCM_TurnIndicatorDig == 0) && (IPM_SensorState == 0) && (FLR_SRR_Obj_Failure == 0) && (FRR_SystemStatus ~= 7) && (RRR_SystemStatus ~= 7) && (RLR_SRR_Obj_Failure == 0)]
    Enable_both -> ACTIVE_R [order 4] : [(ADU1_TurnLightReq == 2) && (BCM_TurnIndicatorDig == 0) && (IPM_SensorState == 0) && (FLR_SRR_Obj_Failure == 0) && (FRR_SystemStatus ~= 7) && (RRR_SystemStatus ~= 7) && (RLR_SRR_Obj_Failure == 0)]
  note: 注释：
      | 1.从Wait_L到Moving_L的Moving_L_Enable_Test是测试用的；（已删除）
      | 2.从Wait_L到End_L的Moving_L_Enable_Test是测试用的；（已删除）
      | 3.从End_L到StandBy的End_L_Finish_Test是测试用的。
      | 4. 2.(after(t_planning, sec)) && (End_L_Finish_Test == 1)改成(after(t_planning, sec)) ---2023.08.31
  note: 注释：
      | 1.从End_R到StandBy的End_R_Finish_Test是测试用的。
      | 2.(after(t_planning, sec)) && (End_R_Finish_Test == 1)改成(after(t_planning, sec)) ---2023.08.31
  (default) -> DCLC_OFF
  DCLC_OFF -> DCLC_ON : [IVI_DCLC_ON == 1]
  DCLC_ON -> DCLC_OFF : [IVI_DCLC_ON ~= 1]
  data: ABS_VehSpdLgt input; ADU1_LongCtrlMode input; ADU1_TurnLightReq input; BCM_TurnIndicatorDig input; Curve_Threshold input; EPS2_EPS1TASTrq input; FLR_SRR_Obj_Failure input; FRR_SystemStatus input; Front_Distance_Threshold input; IPM_LeftLine_Color input; IPM_LeftLine_Type input; IPM_LeftLine_dy input; IPM_LeftLine_hor_curve input; IPM_RightLine_dy input; IPM_SensorState input; K_LCD_Wait_Time_Low input; K_LCD_Wait_Time_Upper input; K_SACC_Override_Time input; Left_Front_Distance_Threshold input; Left_Line_Width_Threshold input; Left_Rear_Distance_Threshold input; MRR_F_Object_dist input; MRR_HWFail input; Negative_Torque input; Positive_Torque input; RLR_OBJ1_Dist input; RLR_SRR_Obj_Failure input; RRR_OBJ1_Dist input; RRR_SystemStatus input; Right_Front_Distance_Threshold input; Right_Line_Width_Threshold input; Right_Rear_Distance_Threshold input; Speed_Max input; Speed_Min input; t_planning input; left_lane_line_clear input; right_lane_line_clear input; FLR_OBJ1_Dist input; FRR_OBJ1_Dist input; DCLC_sts output; IVI_DCLC_ON input; Reach_Destination input; ACC_Enable input; LKA_Enable input; IPM_RightLine_Color input; IPM_RightLine_Type input; IPM_RightLine_hor_curve input; Pass_Midline input

== matlab function ALL_JP360_DBW_V6_5_1103/DCLC1/DCLC状态机/MATLAB Function ==
  data: v_m_s output; vx input; v_km_h output; vy input
function [v_m_s, v_km_h] = fcn(vx, vy)

v_km_h = sqrt(vx * vx + vy * vy);
v_m_s = v_km_h / 3.6;

== matlab function ALL_JP360_DBW_V6_5_1103/ACC_Control/ACC_FUNCTION/Subsystem2/ACC_model/TIS1 ACC action/Subsystem1/mode change/cc and close and follow/cc and close/move close/MATLAB Function2 ==
  data: delta_v input; acc output; dx input; a_dem input; dec output; a_close input; cc_throttle input; cc_brake input
function [acc, dec] = fcn(delta_v, dx, a_dem, a_close, cc_throttle, cc_brake)
    if delta_v * delta_v / (single(2)*a_dem) + single(4) >= dx
        acc = single(0);
        dec = a_close;
    else
        acc = cc_throttle;
        dec = cc_brake;
    end
end

== matlab function ALL_JP360_DBW_V6_5_1103/CIPV1/Lane Line Construction1/Embedded MATLAB Function1 ==
  data: R input; line_data output; SteerWheelAngle input
function line_data = line_count_fun(R, SteerWheelAngle)
if R>100
    line_data = single([1.875, 0, 0, 0]);
else
    if SteerWheelAngle < 0  %turn right
        IPM_Line_C0 = 1.875;
        IPM_Line_C1 = 0;
        IPM_Line_C2 = -(1/(R+1.875));
        line_data = single([IPM_Line_C0, IPM_Line_C1, IPM_Line_C2, 0]);
    else
        IPM_Line_C0 = 1.875;
        IPM_Line_C1 = 0;
        IPM_Line_C2 = 1/(R-1.875);
        line_data = single([IPM_Line_C0, IPM_Line_C1, IPM_Line_C2, 0]);
    end
end
end

== matlab function ALL_JP360_DBW_V6_5_1103/CIPV1/Lane Line Construction1/Embedded MATLAB Function10 ==
  data: IPM_Line_Existence_Probability input; IPM_Line_C0 input; judge_cover_line output; IPM_Line_C1 input; IPM_Line_C2 input; IPM_Line_C3 input
function judge_cover_line = line_fun(IPM_Line_Existence_Probability, IPM_Line_C0, IPM_Line_C1, IPM_Line_C2, IPM_Line_C3)
x = 4.174;
y = -1.083;
if IPM_Line_Existence_Probability >= 0.5
    y_ = IPM_Line_C0 + IPM_Line_C1*x + IPM_Line_C2/2*x^2 + IPM_Line_C3/6*x^3;  %判断是否压线
    if y_>y   %压线
        judge_cover_line = 1;
    else
        judge_cover_line = 0;

    end
else
    judge_cover_line = 1;
end

== matlab function ALL_JP360_DBW_V6_5_1103/CIPV1/Lane Line Construction1/Embedded MATLAB Function2 ==
  data: judge output; IPM_Line_Existence_Probability input; IPM_Line_C0 input; line_data output; IPM_Line_C1 input; IPM_Line_C2 input; IPM_Line_C3 input; judge_cover_line_left input; judge_cover_line_right input
function [judge, line_data]  = line_fun(IPM_Line_Existence_Probability, IPM_Line_C0, IPM_Line_C1, IPM_Line_C2, IPM_Line_C3, judge_cover_line_left, judge_cover_line_right)


if IPM_Line_Existence_Probability >= 0.5 && judge_cover_line_left==0 && judge_cover_line_right==0 
    line_data = single([IPM_Line_C0, IPM_Line_C1, IPM_Line_C2, IPM_Line_C3]);
    judge = 1;
else
    line_data = single([0,0,0,0]);
    judge = 0;
end
end

== matlab function ALL_JP360_DBW_V6_5_1103/DCLC1/DCLC状态机/MATLAB Function2 ==
  data: left_line_type input; vleft_line_type output; leftleft_line_pro input
function vleft_line_type = fcn(left_line_type, leftleft_line_pro)

% left_line_type 左车道线类型，3 表示虚线
% 0x0: Undecided
% 0x1: Solid实线
% 0x2: Road Edge道路边缘
% 0x3: Dashed虚线
% 0x4: Double 双线
% 0x5: Bott's Dots美国特有的凸点标线
% leftleft_line_pro 左左车道线置信度

if (left_line_type == 3) && (leftleft_line_pro > 0.7)
    vleft_line_type = 3;
else
    vleft_line_type = 1;
end

== matlab function ALL_JP360_DBW_V6_5_1103/DCLC1/DCLC状态机/MATLAB Function3 ==
  data: right_line_type input; vright_line_type output; rightright_line_pro input
function vright_line_type = fcn(right_line_type, rightright_line_pro)

% right_line_type 右车道线类型，3 表示虚线
% 0x0: Undecided
% 0x1: Solid实线
% 0x2: Road Edge道路边缘
% 0x3: Dashed虚线
% 0x4: Double 双线
% 0x5: Bott's Dots美国特有的凸点标线
% leftleft_line_pro 左左车道线置信度

if (right_line_type == 3) && (rightright_line_pro > 0.7)
    vright_line_type = 3;
else
    vright_line_type = 1;
end

== matlab function ALL_JP360_DBW_V6_5_1103/CIPV1/Lane Line Construction1/Embedded MATLAB Function3 ==
  data: R input; SteerWheelAngle input; line_data output
function line_data = line_count_fun(R, SteerWheelAngle)
if R>100
    line_data = single([-1.875, 0, 0, 0]);
else
    if SteerWheelAngle < 0  %turn right
        IPM_Line_C0 = -1.875;
        IPM_Line_C1 = 0;
        IPM_Line_C2 = -(1/(R-1.875));
        line_data = single([IPM_Line_C0, IPM_Line_C1, IPM_Line_C2, 0]);
    else
        IPM_Line_C0 = -1.875;
        IPM_Line_C1 = 0;
        IPM_Line_C2 = 1/(R+1.875);
        line_data = single([IPM_Line_C0, IPM_Line_C1, IPM_Line_C2, 0]);
    end
end
end

== matlab function ALL_JP360_DBW_V6_5_1103/CIPV1/Lane Line Construction1/Embedded MATLAB Function4 ==
  data: judge output; IPM_Line_Existence_Probability input; IPM_Line_C0 input; line_data output; IPM_Line_C1 input; IPM_Line_C2 input; IPM_Line_C3 input; judge_cover_line_left input; judge_cover_line_right input
function [judge, line_data] = line_fun(IPM_Line_Existence_Probability, IPM_Line_C0, IPM_Line_C1, IPM_Line_C2, IPM_Line_C3, judge_cover_line_left, judge_cover_line_right)

if IPM_Line_Existence_Probability >= 0.5 && judge_cover_line_left==0 && judge_cover_line_right==0
    line_data = single([IPM_Line_C0, IPM_Line_C1, IPM_Line_C2, IPM_Line_C3]);
    judge = 1;
else
    line_data = single([0, 0, 0, 0]);
    judge = 0;

end
end

== matlab function ALL_JP360_DBW_V6_5_1103/DCLC1/DCLC状态机/计算与前车安全距离 ==
  data: ego_speed input; L2S output; ego_acc input; obs_speed input; t_headway input; t_del input; t_lc input
function L2S = fcn(ego_speed, ego_acc, obs_speed, t_headway, t_del, t_lc)
if ego_speed >= obs_speed
%     L2S = (ego_speed - obs_speed)*(t_lc + t_del) + (ego_speed - obs_speed)^2 / (2 * ego_acc) + ego_speed * t_headway;
    L2S = (ego_speed - obs_speed)*(t_lc + t_del) + ego_speed * t_headway;
else
%     L2S = (ego_speed - obs_speed)*(t_lc + t_del) - (ego_speed - obs_speed)^2 / (2 * ego_acc) + ego_speed * t_headway;
    L2S = (ego_speed - obs_speed)*(t_lc + t_del) + ego_speed * t_headway;
end

== matlab function ALL_JP360_DBW_V6_5_1103/DCLC1/DCLC状态机/计算与右前车安全距离 ==
  data: ego_speed input; L2S output; ego_acc input; obs_speed input; t_headway input; t_del input; t_lc input
function L2S = fcn(ego_speed, ego_acc, obs_speed, t_headway, t_del, t_lc)
if ego_speed >= obs_speed
    L2S = (ego_speed - obs_speed)*(t_lc + t_del) + ego_speed * t_headway;
else
    L2S = (ego_speed - obs_speed)*(t_lc + t_del) + ego_speed * t_headway;
end

== matlab function ALL_JP360_DBW_V6_5_1103/DCLC1/DCLC状态机/计算与右后车安全距离 ==
  data: ego_speed input; L2S output; ego_acc input; obs_speed input; t_headway input; t_del input; t_lc input
function L2S = fcn(ego_speed, ego_acc, obs_speed, t_headway, t_del, t_lc)
if ego_speed >= obs_speed
    L2S = (ego_speed - obs_speed)*(t_lc + t_del) + ego_speed * t_headway;
else
    L2S = (ego_speed - obs_speed)*(t_lc + t_del) + ego_speed * t_headway;
end

== matlab function ALL_JP360_DBW_V6_5_1103/DCLC1/DCLC状态机/计算与左前车安全距离 ==
  data: ego_speed input; L2S output; ego_acc input; obs_speed input; t_headway input; t_del input; t_lc input
function L2S = fcn(ego_speed, ego_acc, obs_speed, t_headway, t_del, t_lc)
if ego_speed >= obs_speed
%     L2S = (ego_speed - obs_speed)*(t_lc + t_del) + (ego_speed - obs_speed)^2 / (2 * ego_acc) + ego_speed * t_headway;
    L2S = (ego_speed - obs_speed)*(t_lc + t_del) + ego_speed * t_headway;
else
%     L2S = (ego_speed - obs_speed)*(t_lc + t_del) - (ego_speed - obs_speed)^2 / (2 * ego_acc) + ego_speed * t_headway;
    L2S = (ego_speed - obs_speed)*(t_lc + t_del) + ego_speed * t_headway;
end

== matlab function ALL_JP360_DBW_V6_5_1103/DCLC1/DCLC状态机/计算与左后车安全距离 ==
  data: ego_speed input; L2S output; ego_acc input; obs_speed input; t_headway input; t_del input; t_lc input
function L2S = fcn(ego_speed, ego_acc, obs_speed, t_headway, t_del, t_lc)
if ego_speed >= obs_speed
    L2S = (ego_speed - obs_speed)*(t_lc + t_del) + ego_speed * t_headway;
else
    L2S = (ego_speed - obs_speed)*(t_lc + t_del) + ego_speed * t_headway;
end

== matlab function ALL_JP360_DBW_V6_5_1103/DCLC1/DCLC状态机/超控判断 ==
  data: u output; brake input; throt input
function u = fcn(brake, throt)
if (brake == 1) || (throt > 90)    %throt 因为维持车速要加油，油门超控暂时修改
    u = 1;
else
    u = 0;
end

== matlab function ALL_JP360_DBW_V6_5_1103/DCLC1/DCLC状态机/车道清晰度判断1 ==
  data: u input; y output
function y = fcn(u)

if u >= single(0.75)
    y = 1;
else
    y = 0;
end

== matlab function ALL_JP360_DBW_V6_5_1103/DCLC1/DCLC状态机/车道清晰度判断2 ==
  data: u input single; y output int8 size=1
function y = fcn(u)

if u >= single(0.75)
    y = int8(1);
else
    y = int8(0);
end
end

== matlab function ALL_JP360_DBW_V6_5_1103/DCLC1/LQR/LQR_offline ==
  data: k1 input; k output; k2 input; k3 input; k4 input; vx input; kappa input; yr input
function k  = fcn(k1,k2,k3,k4,vx, kappa, yr)
  v = abs(vx);
  if v < 0.01
      k=[0,0,0,0];
      return;
%   elseif v <= 11.5
%       k4 = 0.2;
  elseif v <= 17.5
      k4 = 0.2;
  elseif v <= 19.5
      k4 = 0.24;
  else
      k4 = 0.27;
  end
%       index = single(round(abs(vx)/0.01));
%       if index >= length(k1)
%           index = single(length(k1));
%       end
  k3 = max(0.3, double(abs(yr)*k4));
%       if abs(kappa) < 1e-3
%           k3 = k3*5;
% %           if abs(yr) < 1
% %               k3 = 2;
% %           end
%       end

      %index = index>length(k1)? length(k1):indix;
%       k=[k1(index), k2(index), k3(index), k4(index)];
  k=[k1, k2, k3, 0];
end

== matlab function ALL_JP360_DBW_V6_5_1103/DCLC1/LQR/MATLAB Function1 ==
  data: k input; lqr_angle output; err input
function lqr_angle = fcn(k,err)
   lqr_angle=k*err;
end

== stateflow chart ALL_JP360_DBW_V6_5_1103/CanbusControl/Subsystem4/Chart ==
  state a1
    data1=0;
  state a2
    data1=1;
  (default) -> a1
  a2 -> a1 : [data~=2&&data~=3&&data~=5&&data~=6]
  a1 -> a2 : [data==2||data==3||data==5||data==6]
  data: data input; data1 output

== stateflow chart ALL_JP360_DBW_V6_5_1103/button/ACCset/Chart1 ==
  settings: executeAtInitialization=1
  state a2
    en:
    TimeGapSet=3;
  state a1
    en:
    TimeGapSet=4;
  state a3
    en:
    TimeGapSet=2;
  state a4
    en:
    TimeGapSet=1;
  (default) -> a1
  a2 -> a3
  a3 -> a4
  a1 -> a2
  a4 -> a1
  data: TimeGapSet output int8
  events: event input RISING_EDGE_EVENT

== stateflow chart ALL_JP360_DBW_V6_5_1103/button/ACCset/accsetv4 ==
  state s1
    speedout=0;
  state s
    speedout=speed;
  (default) -> s1
  s1 -> s : [accs==3]
  s -> s1 : [accs~=3]
  data: speedout output int8; accs input; speed input
